simulink model "UAM_Flight_control"  (R2024b)
settings: Solver=FixedStepAuto  StartTime=0.0  StopTime=inf  RelTol=1e-3  EnableMultiTasking=on
undefined symbols (not defined in the file): CityMission, control, controlParams, ControlSampleTime, Cruise_a, DiscIntNeverNeededParam, Earth, FixedWingMission, flightState, FSState, FWControlParams, FWTrimSpeed, HoverMission, params, position, R_WAYPOINTTRANSITION, TransitionMission, uavParam, Vt, w_trim, WGS84, zGround
libraries: slpidlib x56, simulink x35, uavalgslib x8, robotcorelib x2, simulink_extras x2, mspfiltlib x1, aerolibtransform2 x1
(part 1 of 12)
settings Model: DataDictionary=UAM_data.sldd  SimulationMode=external  ExtModeTrigDurationFloating=inf  Creator=admin  LastModifiedBy=USER
settings SolverCC: PositivePriorityOrder=on  AutoInsertRateTranBlk=on
settings OptimizationCC: EnhancedBackFolding=on  PassReuseOutputArgsAs=Individual arguments  ZeroExternalMemoryAtStartup=off  ZeroInternalMemoryAtStartup=off  MaxStackSize=500000  OptimizeBlockOrder=speed  DifferentSizesBufferReuse=on  OptimizationCustomize=off  EfficientTunableParamExpr=on
settings DebuggingCC: ParameterTunabilityLossMsg=error
settings HardwareCC: ProdBitPerLong=64  ProdLargestAtomicInteger=LongLong  ProdLargestAtomicFloat=Double  ProdLongLongMode=on  ProdHWDeviceType=ARM Compatible->ARM Cortex-A (64-bit)
settings ModelReferenceCC: ModelReferenceNumInstancesAllowed=Single
settings SFSimCC: MATLABDynamicMemAlloc=off
settings RTWCC: Description=Embedded Coder  SystemTargetFile=ert.tlc  TemplateMakefile=ert_default_tmf  Toolchain=Linaro AArch64 Linux v6.3.1
settings CodeAppCC: ForceParamTrailComments=on  IgnoreCustomStorageClasses=off  OperatorAnnotations=on  SimulinkDataObjDesc=on  SFDataObjDesc=on  InsertBlockDesc=on
settings ERTTargetCC: TargetLangStandard=C99 (ISO)  ExtModeTransport=1  ExtModeMexFile=ext_serial_win32_comm  InlinedParameterPlacement=Hierarchical  ERTCustomFileTemplate=example_file_process.tlc

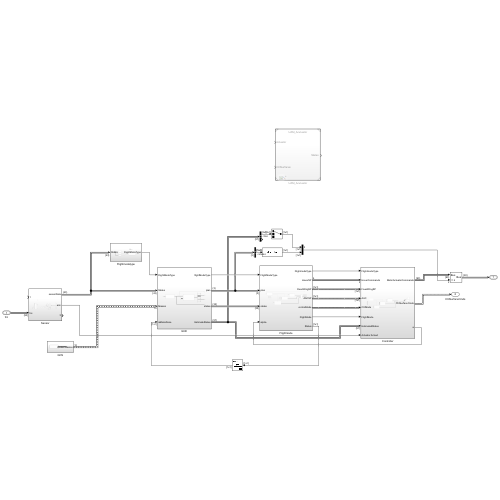
[thumbnail: Simulink's stored preview of the top-level diagram]
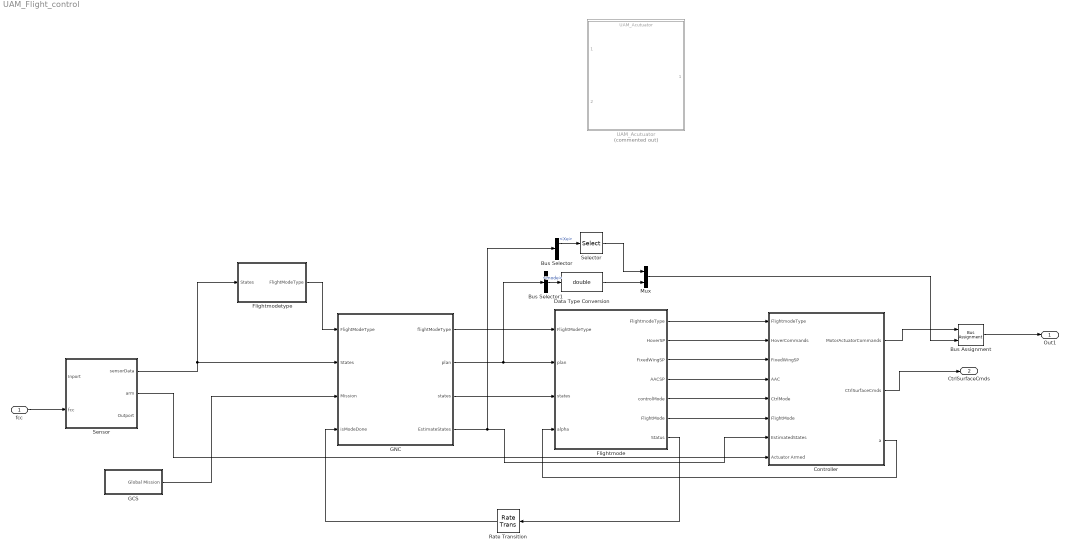
== system UAM_Flight_control ==
  fcc : Inport  OutDataTypeStr=Bus: FCCData
  Bus Assignment : BusAssignment  AssignedSignals=z
  Bus Selector : BusSelector  OutputSignals=Xe,Ve
  Bus Selector1 : BusSelector  OutputSignals=mode
  Controller : Subsystem
  Data Type Conversion : DataTypeConversion  OutDataTypeStr=double  SaturateOnIntegerOverflow=off  RndMeth=Floor
  Flightmode : Subsystem
  Flightmodetype : Subsystem
  GCS : Subsystem
  GNC : Subsystem
  Mux : Mux  Inputs=2
  Rate Transition : RateTransition
  Selector : Selector  InputPortWidth=3  IndexOptions=Index vector (dialog)  Indices=1  OutputSizes=1
  Sensor : Subsystem
  UAM_Acutuator : ModelReference  Commented=on  ModelNameDialog=UAM_Acutuator.slx  SimulationMode=Normal  ModelReferenceVersion=1.21
  Out1 : Outport  OutDataTypeStr=Bus: FCCData  VectorParamsAs1DForOutWhenUnconnected=off
  CtrlSurfaceCmds : Outport  Port=2
  wires:
  Sensor/1(sensorData) -> Flightmodetype/1(States), GNC/2(States)
  GCS/1(Global Mission) -> GNC/3(Mission)
  Flightmodetype/1(FlightModeType) -> GNC/1(FlightModeType)
  GNC/1(flightModeType) -> Flightmode/1(FlightModeType)
  GNC/2(plan) -> Bus Selector1/1, Flightmode/2(plan)
  GNC/3(states) -> Flightmode/3(states)
  Flightmode/1(FlightmodeType) -> Controller/1(FlightmodeType)
  Flightmode/2(HoverSP) -> Controller/2(HoverCommands)
  Flightmode/3(FixedWingSP) -> Controller/3(FixedWingSP)
  Flightmode/4(AACSP) -> Controller/4(AAC)
  Flightmode/5(controlMode) -> Controller/5(CtrlMode)
  Flightmode/6(FlightMode) -> Controller/6(FlightMode)
  GNC/4(EstimateStates) -> Bus Selector/1, Controller/7(EstimatedStates)
  Flightmode/7(Status) -> Rate Transition/1
  Rate Transition/1 -> GNC/4(isModeDone)
  Sensor/2(arm) -> Controller/8(Actuator Armed)
  fcc/1 -> Sensor/2(fcc)
  Controller/3(a) -> Flightmode/4(alpha)
  Controller/2(CtrlSurfaceCmds) -> CtrlSurfaceCmds/1
  Bus Assignment/1 -> Out1/1
  Controller/1(MotorActuatorCommands) -> Bus Assignment/1
  Bus Selector/1 -> Selector/1  "<Xe>"
  Bus Selector1/1 -> Data Type Conversion/1  "<mode>"
  Data Type Conversion/1 -> Mux/2
  Mux/1 -> Bus Assignment/2
  Selector/1 -> Mux/1

== system UAM_Flight_control/Controller ==
  FlightmodeType : Inport  OutDataTypeStr=Enum: FlightModeType
  HoverCommands : Inport  Port=2  OutDataTypeStr=Bus: HoverSPBus
  FixedWingSP : Inport  Port=3  OutDataTypeStr=Bus: FixedWingCommandBus
  AAC : Inport  Port=4  OutDataTypeStr=Bus: AAC
  CtrlMode : Inport  Port=5  OutDataTypeStr=Bus: controlMode
  FlightMode : Inport  Port=6
  EstimatedStates : Inport  Port=7  OutDataTypeStr=Bus: StateBus
  Actuator Armed : Inport  Port=8
  Auto1 : Subsystem  TreatAsAtomicUnit=on
  Bus Selector : BusSelector  OutputSignals=MotorActuatorCommands,CtrlSurfaceCommands,a
  Bus Selector1 : BusSelector  OutputSignals=m
  Bus Selector2 : BusSelector  OutputSignals=rpy_sp
  Display : Display
  Display1 : Display
  Emergency : Subsystem  TreatAsAtomicUnit=on
  Manual : Subsystem  TreatAsAtomicUnit=on
  Merge : Merge  Inputs=3
  Switch Case : SwitchCase  CaseConditions={FlightModeType.Manual, FlightModeType.Auto, FlightModeType.Emergecny}  ShowDefaultCase=off
  MotorActuatorCommands : Outport  OutDataTypeStr=Bus: FCCData
  CtrlSurfaceCmds : Outport  Port=2  OutDataTypeStr=Bus: FixedWingCtrlBus
  a : Outport  Port=3
  wires:
  Bus Selector/3 -> a/1  "<a>"
  [CtrlMode] -> Emergency/1(CtrlMode)
  [CtrlMode] -> Manual/2(CtrlMode)
  AAC/1 -> [AAC]
  [CtrlMode] -> Auto1/4(CtrlMode)
  [FlightMode] -> Emergency/2(FlightMode)
  [EstimatedStates] -> Auto1/6(EstimatedStates)
  Actuator Armed/1 -> [Armed]
  Switch Case/2 -> Auto1/Action
  Bus Selector/2 -> CtrlSurfaceCmds/1  "<CtrlSurfaceCommands>"
  FlightmodeType/1 -> Switch Case/1
  Bus Selector1/1 -> Display/1  "<m>"
  [AAC] -> Auto1/3(AAC)
  CtrlMode/1 -> [CtrlMode]
  Manual/1(Controller) -> Merge/1
  Bus Selector/1 -> Bus Selector2/1, Bus Selector1/1, MotorActuatorCommands/1  "<MotorActuatorCommands>"
  Auto1/1(Controller) -> Merge/2
  Emergency/1(Controller) -> Merge/3
  Switch Case/3 -> Emergency/Action
  Switch Case/1 -> Manual/Action
  [EstimatedStates] -> Manual/4(EstimatedStates)
  [Armed] -> Manual/5(Actuator Armed)
  [FixedWingSP] -> Auto1/2(FixedWingSP)
  FlightMode/1 -> [FlightMode]
  [FlightMode] -> Manual/3(FlightMode)
  FixedWingSP/1 -> [FixedWingSP]
  HoverCommands/1 -> [HoverCommands]
  [EstimatedStates] -> Emergency/3(EstimatedStates)
  [HoverCommands] -> Auto1/1(HoverCommands)
  [Armed] -> Emergency/4(Actuator Armed)
  EstimatedStates/1 -> [EstimatedStates]
  [FlightMode] -> Auto1/5(FlightMode)
  [Armed] -> Auto1/7(" Armed")
  [HoverCommands] -> Manual/1(HoverConmmands)
  Merge/1 -> Bus Selector/1
  Bus Selector2/1 -> Display1/1  "<rpy_sp>"

== system UAM_Flight_control/Flightmode ==
  FlightModeType : Inport
  plan : Inport  Port=2  OutDataTypeStr=Bus: plan
  states : Inport  Port=3  OutDataTypeStr=Bus: states
  alpha : Inport  Port=4
  Auto : Subsystem  TreatAsAtomicUnit=on
  Bus Selector : BusSelector  OutputSignals=HoverSP,FixedWingSP,AACSP,controlMode,FlightMode,Status
  Emergency : Subsystem  TreatAsAtomicUnit=on
  Manual : Subsystem  TreatAsAtomicUnit=on
  Merge : Merge  Inputs=3
  Rate Transition{,1..7} (8 alike) : RateTransition
  Switch Case : SwitchCase  CaseConditions={FlightModeType.Manual, FlightModeType.Auto, FlightModeType.Emergecny}  ShowDefaultCase=off
  Unit Delay : UnitDelay  SampleTime=-1  HasFrameUpgradeWarning=on
  Unit Delay1 : UnitDelay  SampleTime=-1  HasFrameUpgradeWarning=on
  Unit Delay2 : UnitDelay  SampleTime=-1  HasFrameUpgradeWarning=on
  FlightmodeType : Outport  OutDataTypeStr=Enum: FlightModeType
  HoverSP : Outport  Port=2  OutDataTypeStr=Bus: HoverSPBus
  FixedWingSP : Outport  Port=3  OutDataTypeStr=Bus: FixedWingCommandBus
  AACSP : Outport  Port=4  OutDataTypeStr=Bus: AAC
  controlMode : Outport  Port=5  OutDataTypeStr=Bus: controlMode
  FlightMode : Outport  Port=6
  Status : Outport  Port=7
  wires:
  Switch Case/1 -> Manual/Action
  Rate Transition2/1 -> AACSP/1
  [states] -> Manual/1(states)
  Bus Selector/1 -> Rate Transition/1  "<HoverSP>"
  Bus Selector/2 -> Rate Transition1/1  "<FixedWingSP>"
  [alpha] -> Emergency/2(alpha)
  Rate Transition/1 -> HoverSP/1
  [states] -> Emergency/1(states)
  Switch Case/3 -> Emergency/Action
  Rate Transition1/1 -> FixedWingSP/1
  Bus Selector/3 -> Rate Transition2/1  "<AACSP>"
  Bus Selector/5 -> Rate Transition4/1  "<FlightMode>"
  [alpha] -> Manual/2(alpha)
  Rate Transition3/1 -> controlMode/1
  Bus Selector/4 -> Rate Transition3/1  "<controlMode>"
  Bus Selector/6 -> Status/1  "<Status>"
  plan/1 -> Unit Delay/1
  Rate Transition4/1 -> FlightMode/1
  FlightModeType/1 -> FlightmodeType/1, Switch Case/1
  Merge/1 -> Bus Selector/1
  [plan] -> Rate Transition7/1
  [states] -> Rate Transition6/1
  [alpha] -> Rate Transition5/1
  Switch Case/2 -> Auto/Action
  alpha/1 -> Unit Delay2/1
  states/1 -> Unit Delay1/1
  Rate Transition6/1 -> Auto/2(states)
  Rate Transition5/1 -> Auto/3(alpha)
  Rate Transition7/1 -> Auto/1(plan)
  Manual/1(FlightMode) -> Merge/1
  Auto/1(FlightMode) -> Merge/2
  Emergency/1(FlightMode) -> Merge/3
  Unit Delay/1 -> [plan]
  Unit Delay1/1 -> [states]
  Unit Delay2/1 -> [alpha]

== system UAM_Flight_control/Flightmodetype ==
  note: 전환조건
      |
      | 1. ManualInput
      | 2. AutoModeRequest
      | 3. Failsafe
  States : Inport  OutDataTypeStr=Bus: sensorData
  Bus Selector : BusSelector  OutputSignals=RC
  Chart1 : Stateflow chart  TreatAsAtomicUnit=on
      settings: PortSchema="{\"entries\":[{\"content\":{\"sides\":[{\"content\":{\"connectorIds\":[\"In2\",\"In3\",\"In1\"]},\"type\":\"ConnectorPlacement.EquallySpacedRectSide\",\"uuid\":\"7f808d98-1a22-47cf-b619-3081c4328c1f\"},{\"content\":{\"connectorIds\":[\"Out1\"],\"side\":\"RIGHT\"},\"type\":\"ConnectorPlacement.EquallySpacedRectSide\",\"uuid\":\"ee1ebc53-214f-4f44-afa8-7e67f94c306f\"},{\"content\":{\"side\":\"TOP\"},\"type\":\"ConnectorPlacement.EquallySpacedRectSide\",\"uuid\":\"a218192b-9bc0-4f77-b8de-414c3f6a9dd6\"}]},\"type\":\"ConnectorPlacement.EquallySpacedConnector\",\"uuid\":\"d7f6b7da-8a65-4043-9f4e-f6645b75040a\"}],\"packageUris\":[\"http://schema.mathworks.com/mf0/Connector/R2020b\"],\"version\":\"1.0\"}"
  Failsafe : Subsystem
  GCS : Subsystem
  RC : Subsystem
  FlightModeType : Outport  OutDataTypeStr=Enum: FlightModeType
  wires:
  States/1 -> Failsafe/1(States), Bus Selector/1
  Chart1/1(mode) -> FlightModeType/1
  RC/1(ManualInput) -> Chart1/2(ManualInput)
  GCS/1(AutoModeRequest) -> Chart1/3(AutoModeRequest)
  Failsafe/1(Failsafe) -> Chart1/1(Failsafe)
  Bus Selector/1 -> GCS/1(RC_input), RC/1(RCInput)  "<RC>"

== system UAM_Flight_control/GCS ==
  Subsystem : Subsystem
  Global Mission : Outport  OutDataTypeStr=Bus: UAVPathManagerBus  SampleTime=0.005  BusOutputAsStruct=on
  wires:
  Subsystem/1(Mission) -> Global Mission/1

== system UAM_Flight_control/GNC ==
  FlightModeType : Inport  OutDataTypeStr=Enum: FlightModeType
  States : Inport  Port=2  OutDataTypeStr=Bus: sensorData
  Mission : Inport  Port=3  OutDataTypeStr=Bus: UAVPathManagerBus  PortDimensions=10  BusOutputAsStruct=on
  isModeDone : Inport  Port=4  OutDataTypeStr=uint8
  Bus Creator : BusCreator  Inputs=3  OutDataTypeStr=Bus: plan
      settings: InheritFromInputs=off
  Bus Creator1 : BusCreator  Inputs=3  OutDataTypeStr=Bus: states
      settings: InheritFromInputs=off
  Bus Selector : BusSelector  OutputSignals=mode,ToWP,FromWP,pose,states,ground
  Guidance : Subsystem
  Navigation : Subsystem
  flightModeType : Outport
  plan : Outport  Port=2  OutDataTypeStr=Bus: plan
  states : Outport  Port=3  OutDataTypeStr=Bus: states
  EstimateStates : Outport  Port=4  OutDataTypeStr=Bus: StateBus
  wires:
  Mission/1 -> Guidance/3(Mission)
  Bus Selector/6 -> Bus Creator1/3  "<ground>"
  Guidance/1(GNCPlan) -> Bus Selector/1
  Bus Selector/3 -> Bus Creator/3  "<FromWP>"
  Bus Selector/1 -> Bus Creator/1  "<mode>"
  FlightModeType/1 -> Guidance/1(mode), flightModeType/1
  Bus Creator1/1 -> states/1
  Bus Selector/4 -> Bus Creator1/1  "<pose>"
  States/1 -> Navigation/1(sensorData)
  isModeDone/1 -> Guidance/4(isModeDone)
  Bus Selector/2 -> Bus Creator/2  "<ToWP>"
  Bus Selector/5 -> Bus Creator1/2  "<states>"
  Bus Creator/1 -> plan/1
  Navigation/1(States) -> EstimateStates/1, Guidance/2(States)

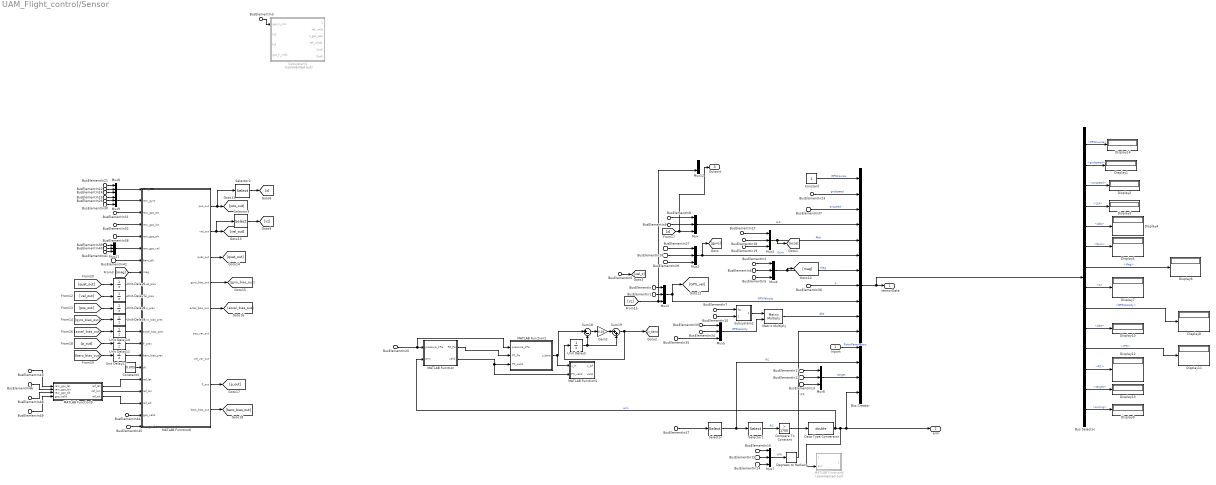
== system UAM_Flight_control/Sensor ==
  Inport : Inport  OutDataTypeStr=Bus: RotorParameters
  BusElementIn14 : Inport  Port=2  PortName=fcc  Element=roll
  BusElementIn15 : Inport  Port=2  PortName=fcc  Element=pitch
  BusElementIn16 : Inport  Port=2  PortName=fcc  Element=yaw
  BusElementIn3 : Inport  Port=2  PortName=fcc  Element=altitude
  BusElementIn8 : Inport  Port=2  PortName=fcc  Element=latitude
  BusElementIn7 : Inport  Port=2  PortName=fcc  Element=latitude
  BusElementIn9 : Inport  Port=2  PortName=fcc  Element=longitude
  BusElementIn10 : Inport  Port=2  PortName=fcc  Element=longitude
  BusElementIn17 : Inport  Port=2  PortName=fcc  Element=acc_x
  BusElementIn18 : Inport  Port=2  PortName=fcc  Element=acc_y
  BusElementIn19 : Inport  Port=2  PortName=fcc  Element=acc_z
  BusElementIn20 : Inport  Port=2  PortName=fcc  Element=pressure
  BusElementIn : Inport  Port=2  PortName=fcc  Element=vel_n
  BusElementIn1 : Inport  Port=2  PortName=fcc  Element=vel_e
  BusElementIn6 : Inport  Port=2  PortName=fcc  Element=vel_d
  BusElementIn23 : Inport  Port=2  PortName=fcc  Element=gndspeed
  BusElementIn11 : Inport  Port=2  PortName=fcc  Element=target_x
  BusElementIn12 : Inport  Port=2  PortName=fcc  Element=target_y
  BusElementIn13 : Inport  Port=2  PortName=fcc  Element=target_z
  BusElementIn27 : Inport  Port=2  PortName=fcc  Element=gyro_x
  BusElementIn28 : Inport  Port=2  PortName=fcc  Element=gyro_y
  BusElementIn29 : Inport  Port=2  PortName=fcc  Element=gyro_z
  BusElementIn2 : Inport  Port=2  PortName=fcc  Element=mag_x
  BusElementIn4 : Inport  Port=2  PortName=fcc  Element=mag_y
  BusElementIn5 : Inport  Port=2  PortName=fcc  Element=mag_z
  BusElementIn33 : Inport  Port=2  PortName=fcc  Element=lin_acc_ecef_x
  BusElementIn34 : Inport  Port=2  PortName=fcc  Element=lin_acc_ecef_y
  BusElementIn35 : Inport  Port=2  PortName=fcc  Element=lin_acc_ecef_z
  BusElementIn36 : Inport  Port=2  PortName=fcc  Element=q
  BusElementIn37 : Inport  Port=2  PortName=fcc  Element=airspeed
  BusElementIn47 : Inport  Port=2  PortName=fcc  Element=rc
  BusElementIn21 : Inport  Port=2  PortName=fcc  Element=raw_acc_x
  BusElementIn22 : Inport  Port=2  PortName=fcc  Element=raw_acc_y
  BusElementIn24 : Inport  Port=2  PortName=fcc  Element=raw_acc_z
  BusElementIn25 : Inport  Port=2  PortName=fcc  Element=raw_gyro_x
  BusElementIn26 : Inport  Port=2  PortName=fcc  Element=raw_gyro_y
  BusElementIn30 : Inport  Port=2  PortName=fcc  Element=raw_gyro_z
  BusElementIn31 : Inport  Port=2  PortName=fcc  Element=raw_gps_lat
  BusElementIn43 : Inport  Port=2  PortName=fcc  Element=raw_gps_lat
  BusElementIn32 : Inport  Port=2  PortName=fcc  Element=raw_gps_lon
  BusElementIn46 : Inport  Port=2  PortName=fcc  Element=raw_gps_lon
  BusElementIn38 : Inport  Port=2  PortName=fcc  Element=raw_gps_alt
  BusElementIn48 : Inport  Port=2  PortName=fcc  Element=raw_gps_alt
  BusElementIn39 : Inport  Port=2  PortName=fcc  Element=raw_vel_n
  BusElementIn40 : Inport  Port=2  PortName=fcc  Element=raw_vel_e
  BusElementIn41 : Inport  Port=2  PortName=fcc  Element=raw_vel_d
  BusElementIn42 : Inport  Port=2  PortName=fcc  Element=baro_alt
  BusElementIn44 : Inport  Port=2  PortName=fcc  Element=gps_valid
  BusElementIn49 : Inport  Port=2  PortName=fcc  Element=gps_valid
  BusElementIn45 : Inport  Port=2  PortName=fcc  Element=baro_valid
  Bus Creator : BusCreator  Inputs=15  OutDataTypeStr=Bus: sensorData
      settings: InheritFromInputs=off
  Bus Selector : BusSelector  OutputSignals=GPSCourse,gndspeed,airspeed,LLA,Abb,Gyro,Mag,q,GPSVelocity,Abe,YPR,RC,target,arming
  Compare To Constant : simulink/Logic and Bit Operations/Compare To Constant  relop=>  const=1700  OutDataTypeStr=boolean
  Constant : Constant
  Constant3 : Constant  Value=0.005
  Data Type Conversion : DataTypeConversion  OutDataTypeStr=double  SaturateOnIntegerOverflow=off  RndMeth=Floor
  Degrees to Radians : simulink_extras/Transformations/Degrees to Radians
  Display{1..14} (14 alike) : Display
  Gain2 : Gain  Gain=0.03
  MATLAB Function : MATLAB Function  TreatAsAtomicUnit=on
  MATLAB Function2 : MATLAB Function  TreatAsAtomicUnit=on
  MATLAB Function5 : MATLAB Function  TreatAsAtomicUnit=on
  MATLAB Function6 : MATLAB Function  Commented=on  TreatAsAtomicUnit=on
  MATLAB Function8 : MATLAB Function  TreatAsAtomicUnit=on  SystemSampleTime=0.005
  MATLAB Function9 : MATLAB Function  TreatAsAtomicUnit=on
  Matrix Multiply : Product  Multiplication=Matrix(*)
  Mux{,1..9,11} (11 alike) : Mux  Inputs=3
  Mux12 : Mux  Inputs=2
  Selector : Selector  InputPortWidth=16  IndexOptions=Index vector (dialog)  Indices=[1:10]  OutputSizes=1
  Selector1 : Selector  InputPortWidth=10  IndexOptions=Index vector (dialog)  Indices=6  OutputSizes=1
  Selector2 : Selector  InputPortWidth=3  IndexOptions=Index vector (dialog)  Indices=3  OutputSizes=1
  Selector3 : Selector  InputPortWidth=3  IndexOptions=Index vector (dialog)  Indices=3  OutputSizes=1
  Subsystem1 : Subsystem  Commented=on
  Subsystem2 : Subsystem
  Sum18 : Sum  Inputs=|+-
  Sum19 : Sum  Inputs=|++
  Unit Delay{6..12} (7 alike) : UnitDelay  SampleTime=-1  HasFrameUpgradeWarning=on
  Unit Delay5 : UnitDelay  SampleTime=0.005  HasFrameUpgradeWarning=on
  sensorData : Outport  OutDataTypeStr=Bus: sensorData
  arm : Outport  Port=2
  Outport : Outport  Port=3
  wires:
  BusElementIn47/1 -> Selector/1
  BusElementIn34/1 -> Mux5/2
  BusElementIn17/1 -> Mux1/1
  Compare To Constant/1 -> Data Type Conversion/1
  Selector/1 -> Bus Creator/13, Selector1/1  "RC"
  BusElementIn4/1 -> Mux4/2
  Subsystem2/1(Out1) -> Matrix Multiply/1
  BusElementIn28/1 -> Mux2/2
  BusElementIn1/1 -> Mux3/2
  BusElementIn9/1 -> Mux/2
  BusElementIn37/1 -> Bus Creator/3  "airspeed"
  BusElementIn35/1 -> Mux5/3
  BusElementIn12/1 -> Mux6/2
  Matrix Multiply/1 -> Bus Creator/10  "Abe"
  BusElementIn27/1 -> Mux2/1
  Selector1/1 -> Compare To Constant/1  "RC"
  Mux5/1 -> Matrix Multiply/2  "GPSVelocity"
  BusElementIn/1 -> Mux3/1
  BusElementIn18/1 -> Mux1/2
  BusElementIn10/1 -> Subsystem2/2(In2)
  BusElementIn36/1 -> Bus Creator/8  "q"
  BusElementIn13/1 -> Mux6/3
  Mux2/1 -> Bus Creator/6, [gyro]  "Gyro"
  BusElementIn7/1 -> Subsystem2/1(fcc)
  Constant/1 -> Bus Creator/1  "GPSCourse"
  BusElementIn2/1 -> Mux4/1
  BusElementIn8/1 -> Mux/1
  Mux/1 -> Bus Creator/4  "LLA"
  BusElementIn33/1 -> Mux5/1
  Data Type Conversion/1 -> MATLAB Function6/2(arm), arm/1, Bus Creator/15, MATLAB Function/2(arm)  "arm"
  Mux4/1 -> [mag], Bus Creator/7  "Mag"
  BusElementIn11/1 -> Mux6/1
  BusElementIn23/1 -> Bus Creator/2  "gndspeed"
  Inport/1 -> Bus Creator/12  "RotorParameters"
  Mux7/1 -> Degrees to Radians/1  "YPR"
  Mux6/1 -> Bus Creator/14  "target"
  BusElementIn16/1 -> Mux7/1
  BusElementIn15/1 -> Mux7/2
  BusElementIn14/1 -> Mux7/3
  Bus Creator/1 -> Bus Selector/1, sensorData/1
  Bus Selector/1 -> Display14/1  "<GPSCourse>"
  Bus Selector/2 -> Display1/1  "<gndspeed>"
  Bus Selector/3 -> Display2/1  "<airspeed>"
  Bus Selector/4 -> Display3/1  "<LLA>"
  Bus Selector/5 -> Display4/1  "<Abb>"
  Bus Selector/6 -> Display5/1  "<Gyro>"
  Bus Selector/7 -> Display6/1  "<Mag>"
  Bus Selector/8 -> Display7/1  "<q>"
  Bus Selector/9 -> Display8/1  "<GPSVelocity>"
  Bus Selector/10 -> Display10/1  "<Abe>"
  Bus Selector/11 -> Display11/1  "<YPR>"
  Bus Selector/12 -> Display12/1  "<RC>"
  Bus Selector/13 -> Display13/1  "<target>"
  Bus Selector/14 -> Display9/1  "<arming>"
  BusElementIn29/1 -> Mux2/3
  BusElementIn5/1 -> Mux4/3
  BusElementIn20/1 -> MATLAB Function2/1(pressure_kPa), MATLAB Function/1(pressure_kPa)
  MATLAB Function/1(P0_Pa) -> MATLAB Function2/2(P0_Pa)
  MATLAB Function/2(valid) -> MATLAB Function5/2(P0_valid), MATLAB Function2/3(P0_valid)
  MATLAB Function2/1(z_baro) -> MATLAB Function5/1(z_in), Sum18/1
  BusElementIn19/1 -> Mux1/3
  Unit Delay5/1 -> Sum19/2, Sum18/2
  Sum18/1 -> Gain2/1
  Gain2/1 -> Sum19/1
  Sum19/1 -> Unit Delay5/1, [z_baro]
  Mux1/1 -> Bus Creator/5, [accel]  "Abb"
  Mux3/1 -> [GPS_vel], Bus Creator/9  "GPSVelocity"
  Degrees to Radians/1 -> Bus Creator/11  "YPR"
  [z] -> Outport/1, Mux/3
  BusElementIn6/1 -> [vel_z]
  [vz] -> Mux12/2, Mux3/3
  BusElementIn21/1 -> Mux8/1
  BusElementIn22/1 -> Mux8/2
  BusElementIn24/1 -> Mux8/3
  Mux8/1 -> MATLAB Function8/1(raw_acc)
  Mux9/1 -> MATLAB Function8/2(raw_gyro)
  BusElementIn25/1 -> Mux9/1
  BusElementIn26/1 -> Mux9/2
  BusElementIn30/1 -> Mux9/3
  BusElementIn31/1 -> MATLAB Function8/3(raw_gps_lat)
  BusElementIn32/1 -> MATLAB Function8/4(raw_gps_lon)
  BusElementIn38/1 -> MATLAB Function8/5(raw_gps_alt)
  BusElementIn39/1 -> Mux11/1
  BusElementIn40/1 -> Mux11/2
  BusElementIn41/1 -> Mux11/3
  Mux11/1 -> MATLAB Function8/6(raw_gps_vel)
  BusElementIn42/1 -> MATLAB Function8/7(baro_alt)
  [mag] -> MATLAB Function8/8(mag)
  BusElementIn44/1 -> MATLAB Function8/20(gps_valid)
  BusElementIn45/1 -> MATLAB Function8/21(baro_valid)
  Constant3/1 -> MATLAB Function8/16(dt)
  Unit Delay6/1 -> MATLAB Function8/9(quat_prev)
  Unit Delay7/1 -> MATLAB Function8/10(vel_prev)
  Unit Delay8/1 -> MATLAB Function8/11(pos_prev)
  Unit Delay9/1 -> MATLAB Function8/12(gyro_bias_prev)
  Unit Delay10/1 -> MATLAB Function8/13(accel_bias_prev)
  Unit Delay11/1 -> MATLAB Function8/14(P_prev)
  Unit Delay12/1 -> MATLAB Function8/15(baro_bias_prev)
  MATLAB Function8/1(pos_out) -> Selector2/1, [pos_out]
  MATLAB Function8/2(vel_out) -> Selector3/1, [vel_out]
  MATLAB Function8/3(quat_out) -> [quat_out]
  MATLAB Function8/4(gyro_bias_out) -> [gyro_bias_out]
  MATLAB Function8/5(accel_bias_out) -> [accel_bias_out]
  MATLAB Function8/8(P_out) -> [p_out]
  MATLAB Function8/9(baro_bias_out) -> [baro_bias_out]
  [vel_out] -> Unit Delay7/1
  [quat_out] -> Unit Delay6/1
  [pos_out] -> Unit Delay8/1
  [gyro_bias_out] -> Unit Delay9/1
  [accel_bias_out] -> Unit Delay10/1
  [p_out] -> Unit Delay11/1
  [baro_bias_out] -> Unit Delay12/1
  MATLAB Function9/1(ref_lat) -> MATLAB Function8/17(ref_lat)
  MATLAB Function9/2(ref_lon) -> MATLAB Function8/18(ref_lon)
  MATLAB Function9/3(ref_alt) -> MATLAB Function8/19(ref_alt)
  BusElementIn43/1 -> MATLAB Function9/1(raw_gps_lat)
  BusElementIn46/1 -> MATLAB Function9/2(raw_gps_lon)
  BusElementIn48/1 -> MATLAB Function9/3(raw_gps_alt)
  BusElementIn49/1 -> MATLAB Function9/4(gps_valid)
  Selector3/1 -> [vz]
  Selector2/1 -> [z]
  BusElementIn3/1 -> Subsystem1/1(gps_h_msl)

== system UAM_Flight_control/Controller/Auto1 ==
  HoverCommands : Inport  OutDataTypeStr=Bus: HoverSPBus
  FixedWingSP : Inport  Port=2
  AAC : Inport  Port=3
  CtrlMode : Inport  Port=4
  FlightMode : Inport  Port=5
  EstimatedStates : Inport  Port=6
  " Armed" : Inport  Port=7
  Action Port : ActionPort  ActionPortLabel=case [ Auto ]:
  Blend Scheduler : Subsystem
  Bus Creator : BusCreator  Inputs=3  OutDataTypeStr=Bus: controller
  Bus Selector2 : BusSelector  OutputSignals=inTransition,TransitionCondition,BackTransitionCondition,TransitionStep
  Fixed Wing Controller : Subsystem  TreatAsAtomicUnit=on  VariantControl=Fixed Wing Controller
  Manual Control : Subsystem
  Multicopter Controller : Subsystem  TreatAsAtomicUnit=on
  Scheduler : Subsystem  SystemSampleTime=0.005
  Controller : Outport
  wires:
  Scheduler/1(MotorActuatorCommands) -> Bus Creator/1  "MotorActuatorCommands"
  Manual Control/1(AERT) -> Fixed Wing Controller/5(AERT)
  Scheduler/2(CtrlSurfaceCommands) -> Bus Creator/2  "CtrlSurfaceCommands"
  Fixed Wing Controller/1(Actuator) -> Scheduler/4(FixedWingActuators)
  Blend Scheduler/2(alpha) -> Bus Creator/3  "a"
  Multicopter Controller/1(MixerCommands) -> Blend Scheduler/3(MixerCommands)
  AAC/1 -> Fixed Wing Controller/3(AAC SP)
  FixedWingSP/1 -> Fixed Wing Controller/4(FixedWingSP)
  [InTransition] -> Multicopter Controller/3(InTransition)
  " Armed"/1 -> Fixed Wing Controller/Enable, Scheduler/Enable, Multicopter Controller/Enable
  HoverCommands/1 -> Multicopter Controller/1(Hover Commands)
  EstimatedStates/1 -> Fixed Wing Controller/1(States), Blend Scheduler/2(States), Multicopter Controller/2(States)
  FlightMode/1 -> Multicopter Controller/5(FlightMode), Blend Scheduler/1(FlightMode)
  Bus Selector2/2 -> [TransitionDone]  "<TransitionCondition>"
  CtrlMode/1 -> Bus Selector2/1, Scheduler/3(CtrlMode), Multicopter Controller/4(CtrlMode), Fixed Wing Controller/2(Control Mode)
  Bus Selector2/1 -> [InTransition]  "<inTransition>"
  Bus Selector2/3 -> [BackTransitionDone]  "<BackTransitionCondition>"
  Bus Creator/1 -> Controller/1
  Blend Scheduler/3(FlightState) -> Scheduler/2(FlightState)
  [InTransition] -> Fixed Wing Controller/6(In1)
  Bus Selector2/4 -> [TransitionStep]  "<TransitionStep>"
  Blend Scheduler/1(MotorCommands) -> Scheduler/1(MotorCommands)

== system UAM_Flight_control/Controller/Emergency ==
  CtrlMode : Inport  OutDataTypeStr=Bus: controlMode
  FlightMode : Inport  Port=2
  EstimatedStates : Inport  Port=3  OutDataTypeStr=Bus: StateBus
  Actuator Armed : Inport  Port=4
  Action Port : ActionPort  ActionPortLabel=case [ Emergecny ]:
  Blend Scheduler : Subsystem
  Bus Creator : BusCreator  Inputs=3  OutDataTypeStr=Bus: controller
  Bus Selector : BusSelector  OutputSignals=TransitionCondition,BackTransitionCondition
  Bus Selector1 : BusSelector  OutputSignals=RC
  Display : Display
  FixedWing Controller : Subsystem  TreatAsAtomicUnit=on  VariantControl=Fixed Wing Controller
  Scheduler : Subsystem  SystemSampleTime=0.005
  multicopter Controller : Subsystem  TreatAsAtomicUnit=on
  Controller : Outport
  wires:
  Blend Scheduler/1(alpha) -> Bus Creator/3, Scheduler/2(BlendingSchedule)  "a"
  [TransitionDone] -> Scheduler/4(TransitionDone)
  EstimatedStates/1 -> FixedWing Controller/1(States), Blend Scheduler/2(States), multicopter Controller/2(States), Bus Selector1/1
  FixedWing Controller/1(Actuator) -> Scheduler/6(FixedWingActuators)
  Bus Selector1/1 -> multicopter Controller/1(RC), FixedWing Controller/3(RC)  "<RC>"
  [BackTransitionDone] -> Scheduler/5(BackTransitionDone)
  Bus Selector/2 -> [BackTransitionDone]  "<BackTransitionCondition>"
  FlightMode/1 -> Blend Scheduler/1(FlightMode)
  Bus Selector/1 -> [TransitionDone]  "<TransitionCondition>"
  Actuator Armed/1 -> Scheduler/Enable, FixedWing Controller/Enable, multicopter Controller/Enable
  CtrlMode/1 -> Bus Selector/1, FixedWing Controller/2(Control Mode)
  Blend Scheduler/2(FlightState) -> Scheduler/3(FlightState)
  multicopter Controller/1(MixerCommands) -> Display/1, Scheduler/1(MotorCommands)
  Scheduler/1(MotorActuatorCommands) -> Bus Creator/1  "MotorActuatorCommands"
  Scheduler/2(CtrlSurfaceCommands) -> Bus Creator/2  "CtrlSurfaceCommands"
  Bus Creator/1 -> Controller/1

== system UAM_Flight_control/Controller/Manual ==
  HoverConmmands : Inport
  CtrlMode : Inport  Port=2  OutDataTypeStr=Bus: controlMode
  FlightMode : Inport  Port=3
  EstimatedStates : Inport  Port=4  OutDataTypeStr=Bus: StateBus
  Actuator Armed : Inport  Port=5
  Action Port : ActionPort  ActionPortLabel=case [ Manual ]:
  Blend Scheduler : Subsystem
  Bus Creator : BusCreator  Inputs=3  OutDataTypeStr=Bus: controller
  Bus Selector : BusSelector  OutputSignals=TransitionCondition,BackTransitionCondition
  Bus Selector1 : BusSelector  OutputSignals=RC
  FixedWing Controller : Subsystem  TreatAsAtomicUnit=on  VariantControl=Fixed Wing Controller
  Scheduler : Subsystem  SystemSampleTime=0.005
  multicopter Controller : Subsystem  TreatAsAtomicUnit=on
  Controller : Outport
  wires:
  Blend Scheduler/1(alpha) -> Bus Creator/3, Scheduler/2(BlendingSchedule)  "a"
  [TransitionDone] -> Scheduler/4(TransitionDone)
  EstimatedStates/1 -> FixedWing Controller/1(States), Blend Scheduler/2(States), multicopter Controller/3(States), Bus Selector1/1
  FixedWing Controller/1(Actuator) -> Scheduler/6(FixedWingActuators)
  Bus Selector1/1 -> FixedWing Controller/3(RC), multicopter Controller/2(RC)  "<RC>"
  [BackTransitionDone] -> Scheduler/5(BackTransitionDone)
  Bus Selector/2 -> [BackTransitionDone]  "<BackTransitionCondition>"
  Bus Selector/1 -> [TransitionDone]  "<TransitionCondition>"
  Actuator Armed/1 -> multicopter Controller/4(arming), Scheduler/Enable, FixedWing Controller/Enable, multicopter Controller/Enable
  CtrlMode/1 -> Bus Selector/1, FixedWing Controller/2(Control Mode)
  Blend Scheduler/2(FlightState) -> Scheduler/3(FlightState)
  multicopter Controller/1(MixerCommands) -> Scheduler/1(MotorCommands)
  Scheduler/1(MotorActuatorCommands) -> Bus Creator/1  "MotorActuatorCommands"
  Scheduler/2(CtrlSurfaceCommands) -> Bus Creator/2  "CtrlSurfaceCommands"
  Bus Creator/1 -> Controller/1
  FlightMode/1 -> Blend Scheduler/1(FlightMode)
  HoverConmmands/1 -> multicopter Controller/1(HoverConmmands)

== system UAM_Flight_control/Flightmode/Auto ==
  plan : Inport  OutDataTypeStr=Bus: plan  SampleTime=0.005
  states : Inport  Port=2  OutDataTypeStr=Bus: states  SampleTime=0.005
  alpha : Inport  Port=3  SampleTime=0.005
  Action Port : ActionPort  ActionPortLabel=case [ Auto ]:
  Bus Creator : BusCreator  Inputs=4  OutDataTypeStr=Bus: HoverSPBus
      settings: InheritFromInputs=off
  Bus Creator1 : BusCreator  Inputs=6  OutDataTypeStr=Bus: flightmode
  Bus Selector : BusSelector  OutputSignals=LAP,YawCmd
  Bus Selector1 : BusSelector  OutputSignals=mode,ToWP,FromWP
  Bus Selector2 : BusSelector  OutputSignals=pose,states,ground
  Compare To Constant : simulink/Logic and Bit Operations/Compare To Constant  relop===  const=2  OutDataTypeStr=boolean
  Constant : Constant  Value=0  OutDataTypeStr=boolean
  Constant2 : Constant  Value=FSState  SampleTime=-1
  Demux : Demux
  Guidance Mode Selector : Stateflow chart  TreatAsAtomicUnit=on
      settings: PortSchema="{\"entries\":[{\"content\":{\"sides\":[{\"content\":{\"connectorIds\":[\"In1\",\"In2\",\"In3\",\"In4\",\"In5\",\"In7\",\"In6\",\"In8\",\"In9\"]},\"type\":\"ConnectorPlacement.EquallySpacedRectSide\",\"uuid\":\"a9cfd0e2-196c-422d-b359-9161a47768c9\"},{\"content\":{\"connectorIds\":[\"Out7\",\"Out2\",\"Out4\",\"Out3\",\"Out5\",\"Out6\",\"Out1\"],\"side\":\"RIGHT\"},\"type\":\"ConnectorPlacement.EquallySpacedRectSide\",\"uuid\":\"4fed41ae-e7cf-4de3-8bdb-9e24e7d8b079\"},{\"content\":{\"side\":\"TOP\"},\"type\":\"ConnectorPlacement.EquallySpacedRectSide\",\"uuid\":\"2d49ff20-2f63-498d-ac9d-820eae01f794\"},{\"content\":{\"side\":\"BOTTOM\"},\"type\":\"ConnectorPlacement.EquallySpacedRectSide\",\"uuid\":\"da24ee44-6e15-4e50-9b36-ff21cb47946d\"}]},\"type\":\"ConnectorPlacement.EquallySpacedConnector\",\"uuid\":\"88d403f4-ad96-40f9-9697-84906f26a8bf\"}],\"packageUris\":[\"http://schema.mathworks.com/mf0/Connector/R2020b\"],\"version\":\"1.0\"}"
  Mux : Mux  Inputs=2
  Stop Simulation : Stop
  Terminator : Terminator
  Unit Delay : UnitDelay  SampleTime=-1  HasFrameUpgradeWarning=on
  FlightMode : Outport  OutDataTypeStr=Bus: flightmode
  wires:
  Bus Selector1/1 -> Guidance Mode Selector/1(mode)  "<mode>"
  Guidance Mode Selector/6(FlightMode) -> Bus Creator1/5  "FlightMode"
  Bus Selector1/3 -> Guidance Mode Selector/3(FromWP)  "<FromWP>"
  Bus Selector2/3 -> Guidance Mode Selector/7(Ground)  "<ground>"
  Bus Selector/1 -> Mux/1  "<LAP>"
  Guidance Mode Selector/5(controlMode) -> Bus Creator1/4  "controlMode"
  Guidance Mode Selector/3(aacSP) -> Bus Creator1/3  "AACSP"
  Guidance Mode Selector/7(InnerLoopCmds) -> Bus Selector/1
  Guidance Mode Selector/2(GdncMode) -> Terminator/1
  Bus Selector/2 -> Mux/2  "<YawCmd>"
  Compare To Constant/1 -> Stop Simulation/1
  Bus Selector2/2 -> Guidance Mode Selector/5(States)  "<states>"
  Mux/1 -> Demux/1
  Bus Selector2/1 -> Guidance Mode Selector/4(Pose)  "<pose>"
  Guidance Mode Selector/1(Status) -> Compare To Constant/1, Bus Creator1/6  "Status"
  Guidance Mode Selector/4(FixedWingSP) -> Bus Creator1/2  "FixedWingSP"
  Bus Selector1/2 -> Guidance Mode Selector/2(ToWP)  "<ToWP>"
  Demux/1 -> Bus Creator/1  "X"
  Demux/2 -> Bus Creator/2  "Y"
  Demux/3 -> Bus Creator/3  "Z"
  Demux/4 -> Bus Creator/4  "Yaw"
  Bus Creator/1 -> Bus Creator1/1  "HoverSP"
  Bus Creator1/1 -> Unit Delay/1
  alpha/1 -> Guidance Mode Selector/8(a)
  Constant2/1 -> Guidance Mode Selector/6(PresetMode)
  states/1 -> Bus Selector2/1
  plan/1 -> Bus Selector1/1
  Unit Delay/1 -> FlightMode/1
  Constant/1 -> Guidance Mode Selector/9(abort_cmd)

== system UAM_Flight_control/Flightmode/Emergency ==
  states : Inport  OutDataTypeStr=Bus: states
  alpha : Inport  Port=2
  Action Port : ActionPort  ActionPortLabel=case [ Emergecny ]:
  Basic Control  Switching : Stateflow chart  TreatAsAtomicUnit=on
  Bus Creator : BusCreator  Inputs=6  OutDataTypeStr=Bus: flightmode
      settings: InheritFromInputs=off
  Bus Creator1 : BusCreator  Inputs=4  OutDataTypeStr=Bus: HoverSPBus
  Bus Selector : BusSelector  OutputSignals=states,states.RC
  Constant{,4..6} (4 alike) : Constant  Value=0
  Constant1 : Constant  Value=struct('roll', 0.0, 'pitch', 0.0, 'yaw', 0.0, 'airspeed', 0.0)  VectorParams1D=off  OutDataTypeStr=Bus: FixedWingCommandBus
  Constant2 : Constant  Value=struct('airspeed', 0.0, 'altitude', 0.0, 'course', 0.0, 'L1', 0.0, 'climbrate', 0.0)  VectorParams1D=off  OutDataTypeStr=Bus: AAC
  Constant3 : Constant  Value=0  OutDataTypeStr=uint8
  Hover : Constant  Value=FSState
  Unit Delay : UnitDelay  SampleTime=-1  HasFrameUpgradeWarning=on
  FlightMode : Outport  OutDataTypeStr=Bus: flightmode
  wires:
  Constant/1 -> Bus Creator1/1  "X"
  Constant5/1 -> Bus Creator1/3  "Z"
  Constant4/1 -> Bus Creator1/2  "Y"
  Basic Control  Switching/2(flightMode) -> Bus Creator/5  "FlightMode"
  Basic Control  Switching/1(controlMode) -> Bus Creator/4  "controlMode"
  Hover/1 -> Basic Control  Switching/1(PresetMode)
  Constant3/1 -> Bus Creator/6  "Status"
  Bus Selector/2 -> Basic Control  Switching/3(trigger)  "<RC>"
  Bus Selector/1 -> Basic Control  Switching/2(States)  "<states>"
  Constant2/1 -> Bus Creator/3  "AACSP"
  alpha/1 -> Basic Control  Switching/4(a)
  Bus Creator1/1 -> Bus Creator/1  "HoverSP"
  states/1 -> Bus Selector/1
  Constant1/1 -> Bus Creator/2  "FixedWingSP"
  Constant6/1 -> Bus Creator1/4  "Yaw"
  Bus Creator/1 -> Unit Delay/1
  Unit Delay/1 -> FlightMode/1

== system UAM_Flight_control/Flightmode/Manual ==
  states : Inport  OutDataTypeStr=Bus: states
  alpha : Inport  Port=2
  Action Port : ActionPort  ActionPortLabel=case [ Manual ]:
  Basic Control  Switching : Stateflow chart  TreatAsAtomicUnit=on
  Bus Creator : BusCreator  Inputs=6  OutDataTypeStr=Bus: flightmode
      settings: InheritFromInputs=off
  Bus Creator1 : BusCreator  Inputs=4  OutDataTypeStr=Bus: HoverSPBus
  Bus Selector : BusSelector  OutputSignals=pose,states,states.RC
  Bus Selector1 : BusSelector  OutputSignals=X,Y,Z,Yaw
  Constant1 : Constant  Value=struct('roll', 0.0, 'pitch', 0.0, 'yaw', 0.0, 'airspeed', 0.0)  VectorParams1D=off  OutDataTypeStr=Bus: FixedWingCommandBus
  Constant2 : Constant  Value=struct('airspeed', 0.0, 'altitude', 0.0, 'course', 0.0, 'L1', 0.0, 'climbrate', 0.0)  VectorParams1D=off  OutDataTypeStr=Bus: AAC
  Constant3 : Constant  Value=0  OutDataTypeStr=uint8
  Display : Display
  Hover : Constant  Value=FSState
  Unit Delay : UnitDelay  SampleTime=-1  HasFrameUpgradeWarning=on
  FlightMode : Outport  OutDataTypeStr=Bus: flightmode
  wires:
  states/1 -> Bus Selector/1
  Basic Control  Switching/2(controlMode) -> Bus Creator/4  "controlMode"
  Hover/1 -> Basic Control  Switching/1(PresetMode)
  Basic Control  Switching/3(flightMode) -> Bus Creator/5  "FlightMode"
  Constant3/1 -> Bus Creator/6  "Status"
  Bus Creator/1 -> Unit Delay/1
  Constant2/1 -> Bus Creator/3  "AACSP"
  Constant1/1 -> Bus Creator/2  "FixedWingSP"
  alpha/1 -> Basic Control  Switching/5(a)
  Bus Selector/2 -> Basic Control  Switching/3(States)  "<states>"
  Bus Selector/3 -> Basic Control  Switching/4(trigger)  "<RC>"
  Unit Delay/1 -> FlightMode/1
  Bus Selector/1 -> Basic Control  Switching/2(pose)  "<pose>"
  Basic Control  Switching/1(HoverSPBUS) -> Bus Selector1/1  "HoverSP"
  Bus Selector1/1 -> Bus Creator1/1  "<X>"
  Bus Selector1/2 -> Bus Creator1/2  "<Y>"
  Bus Selector1/3 -> Bus Creator1/3  "<Z>"
  Bus Selector1/4 -> Bus Creator1/4  "<Yaw>"
  Bus Creator1/1 -> Display/1, Bus Creator/1

== system UAM_Flight_control/Flightmodetype/Failsafe ==
  States : Inport
  Constant : Constant  Value=0
  Data Type Conversion : DataTypeConversion  OutDataTypeStr=boolean  SaturateOnIntegerOverflow=off  RndMeth=Floor
  Failsafe : Outport  OutDataTypeStr=boolean  PortDimensions=1
  wires:
  Constant/1 -> Data Type Conversion/1
  Data Type Conversion/1 -> Failsafe/1

== system UAM_Flight_control/Flightmodetype/GCS ==
  RC_input : Inport
  Compare To Constant : simulink/Logic and Bit Operations/Compare To Constant  relop=>  const=1700  OutDataTypeStr=boolean
  Selector : Selector  InputPortWidth=10  IndexOptions=Index vector (dialog)  Indices=7  OutputSizes=1
  AutoModeRequest : Outport  OutDataTypeStr=boolean
  wires:
  RC_input/1 -> Selector/1
  Selector/1 -> Compare To Constant/1
  Compare To Constant/1 -> AutoModeRequest/1

== system UAM_Flight_control/Flightmodetype/RC ==
  RCInput : Inport
  Compare To Constant : simulink/Logic and Bit Operations/Compare To Constant  relop=<  const=1300  OutDataTypeStr=boolean
  Selector : Selector  InputPortWidth=10  IndexOptions=Index vector (dialog)  Indices=7  OutputSizes=1
  ManualInput : Outport  OutDataTypeStr=boolean
  wires:
  RCInput/1 -> Selector/1
  Compare To Constant/1 -> ManualInput/1
  Selector/1 -> Compare To Constant/1

== system UAM_Flight_control/GCS/Subsystem ==
  note: uavPathManagerBus type
  Airspeed : Constant  Value=16
  Altitude : Constant  Value=0
  Bus Assignment : BusAssignment  AssignedSignals=position,params
  Course : Constant  Value=0
  Flight Mode : Constant  Value=0
  Mux : Mux  Inputs=3
  Mux1 : Mux
  No Mission : Constant  Value=struct('mode',0,'position',[0 0 0]','params',[0;0;0;0]);  OutDataTypeStr=Bus: UAVPathManagerBus
  Variant Source : VariantSource  ShowConditionOnBlock=on
  Waypoints : Constant  Value=FixedWingMission  OutDataTypeStr=Bus: UAVPathManagerBus  SampleTime=-1
  Waypoints1 : Constant  Value=HoverMission  OutDataTypeStr=Bus: UAVPathManagerBus  SampleTime=-1
  Waypoints2 : Constant  Value=TransitionMission  OutDataTypeStr=Bus: UAVPathManagerBus  SampleTime=-1
  Waypoints3 : Constant  Value=CityMission  OutDataTypeStr=Bus: UAVPathManagerBus  SampleTime=-1
  X : Constant  Value=0
  Y : Constant  Value=0
  Z : Constant  Value=10
  Mission : Outport
  wires:
  Waypoints1/1 -> Variant Source/3
  Airspeed/1 -> Mux1/2
  Y/1 -> Mux/2
  No Mission/1 -> Bus Assignment/1
  Z/1 -> Mux/3
  Bus Assignment/1 -> Variant Source/1
  Waypoints/1 -> Variant Source/2
  Flight Mode/1 -> Mux1/1
  X/1 -> Mux/1
  Course/1 -> Mux1/4
  Waypoints3/1 -> Variant Source/5
  Mux/1 -> Bus Assignment/2
  Waypoints2/1 -> Variant Source/4
  Altitude/1 -> Mux1/3
  Mux1/1 -> Bus Assignment/3
  Variant Source/1 -> Mission/1

== system UAM_Flight_control/GNC/Guidance ==
  mode : Inport
  States : Inport  Port=2
  Mission : Inport  Port=3  OutDataTypeStr=Bus: UAVPathManagerBus
  isModeDone : Inport  Port=4
  Atan2 : Trigonometry  Operator=atan2
  Auto : Subsystem  TreatAsAtomicUnit=on
  Bus Selector : BusSelector  OutputSignals=x,y,z,vy,vx
  Emergency : Subsystem  TreatAsAtomicUnit=on
  Merge : Merge  Inputs=3
  Mux : Mux
  Mux1 : Mux  Inputs=2
  Switch Case : SwitchCase  CaseConditions={FlightModeType.Manual, FlightModeType.Auto, FlightModeType.Emergecny}  ShowDefaultCase=off
  Switch Case Action Subsystem : Subsystem  TreatAsAtomicUnit=on
  UAM POS : Subsystem
  UAM States : Subsystem
  ground : Constant  Value=0
  GNCPlan : Outport  OutDataTypeStr=Bus: GNCplan
  wires:
  [pose] -> Emergency/1(pose)
  UAM POS/1(POS) -> Bus Selector/1
  [ground] -> Auto/6(Ground)
  [states] -> Switch Case Action Subsystem/2(states)
  Bus Selector/1 -> Mux/1  "<x>"
  [pose] -> Auto/1(Pose)
  [states] -> Emergency/2(states)
  [isModeDone] -> Auto/3(isModeDone)
  Emergency/1(GNCPlan) -> Merge/3
  [ground] -> Switch Case Action Subsystem/3(ground)
  Auto/1(GNCPlan) -> Merge/2
  [ground] -> Emergency/3(ground)
  Switch Case/1 -> Switch Case Action Subsystem/Action
  Bus Selector/2 -> Mux/2  "<y>"
  [Mission] -> Auto/2(Mission)
  Switch Case Action Subsystem/1(GNCPlan) -> Merge/1
  Atan2/1 -> Mux1/1, Mux/4  "yaw"
  ground/1 -> [ground]
  Merge/1 -> GNCPlan/1
  Switch Case/3 -> Emergency/Action
  [Landingstates] -> Auto/4(LandingStates)
  [states] -> Auto/5(States)
  Bus Selector/3 -> Mux1/2, Mux/3  "<z>"
  [pose] -> Switch Case Action Subsystem/1(pose)
  Switch Case/2 -> Auto/Action
  States/1 -> UAM States/1(UAMStates), UAM POS/1(UAMStates)
  Bus Selector/4 -> Atan2/1  "<vy>"
  Bus Selector/5 -> Atan2/2  "<vx>"
  Mission/1 -> [Mission]
  isModeDone/1 -> [isModeDone]
  UAM States/1(States) -> [states]
  Mux1/1 -> [Landingstates]
  Mux/1 -> [pose]
  mode/1 -> Switch Case/1

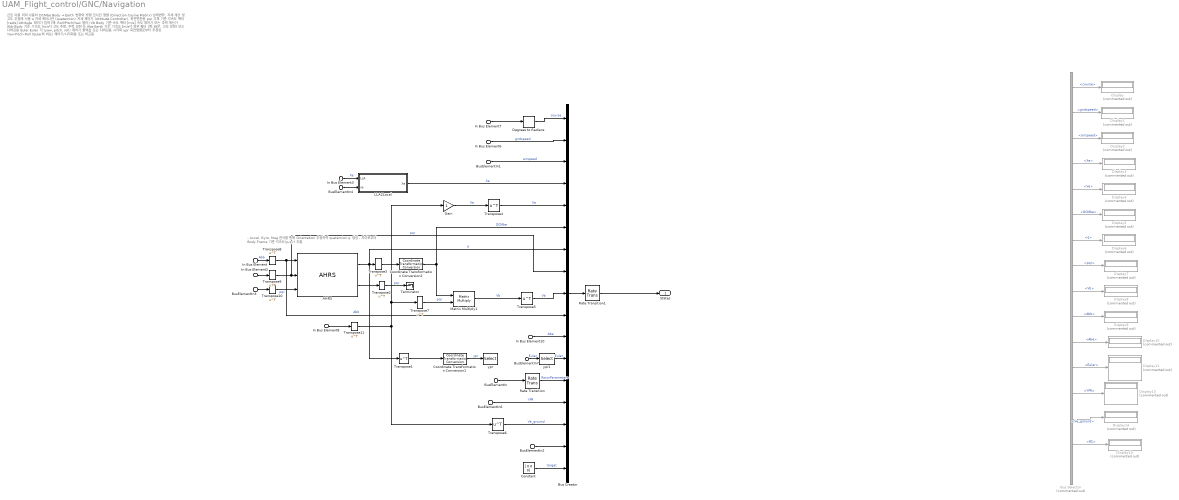
== system UAM_Flight_control/GNC/Navigation ==
  note: 신호 이름
      | 의미
      | 사용처
      |
      | DCMbe
      | Body → Earth 방향의 방향 코사인 행렬 (Direction Cosine Matrix)
      | 상태변환, 자세 계산 및 고도 추정에 사용
      |
      | q
      | 자세 쿼터니언 (quaternion)
      | 자세 제어기 (Attitude Controller), 회전변환용
      |
      | pqr
      | 기체 기준 각속도 벡터 [rad/s]
      | Attitude 제어기 입력 (예: Roll/Pitch/Yaw 제어)
      |
      | Vb
      | Body 기준 속도 벡터 [m/s]
      | 속도 제어기 또는 추력 계산기
      |
      | Abb
      | Body 기준 가속도 [m/s²]
      | 고도 추정, 추력 보정 등
      |
      | Abe
      | Earth 기준 가속도 [m/s²]
      | 외부 필터 (예: EKF, 고도 보정) 또는 디버깅용
      |
      | Euler
      | Euler 각 (yaw, pitch, roll)
      | 제어기 출력값 또는 디버깅용 시각화
      |
      | ypr
      | 회전행렬로부터 추정된 Yaw-Pitch-Roll (Euler와 비슷)
      | 제어기/시각화용 또는 비교용
  note: - Accel, Gyro, Mag 센서를 통해 Orientation 추정하여 quaternion q 생성
      | - 자이로부터 Body Frame 기준 각속도(p,q,r) 추출
  In Bus Element : Inport  PortName=sensorData  Element=Abb
  In Bus Element2 : Inport  PortName=sensorData  Element=Gyro
  In Bus Element3 : Inport  PortName=sensorData  Element=LLA
  In Bus Element6 : Inport  PortName=sensorData  Element=gndspeed
  In Bus Element7 : Inport  PortName=sensorData  Element=GPSCourse
  In Bus Element8 : Inport  PortName=sensorData  Element=GPSVelocity
  In Bus Element10 : Inport  PortName=sensorData  Element=Abe
  BusElementIn : Inport  PortName=sensorData  Element=RotorParameters
  BusElementIn1 : Inport  PortName=sensorData  Element=airspeed
  BusElementIn2 : Inport  PortName=sensorData  Element=RC
  BusElementIn3 : Inport  PortName=sensorData  Element=Mag
  BusElementIn4 : Inport  PortName=sensorData  Element=arming
  BusElementIn6 : Inport  PortName=sensorData  Element=YPR
  BusElementIn7 : Inport  PortName=sensorData  Element=YPR
  AHRS : mspfiltlib/AHRS  DispRefFrame=NED  DecimationFactor=1  InitialProcessNoise=ahrsfilter.defaultProcessNoise  OrientationFormat=quaternion  SimulateUsing=Interpreted execution  AccelerometerNoise=0.0001924722  GyroscopeNoise=9.1385e-5  MagnetometerNoise=0.1  GyroscopeDriftNoise=3.0462e-13  LinearAccelerationNoise=0.0096236100000000012  MagneticDisturbanceNoise=0.5  LinearAccelerationDecayFactor=0.5  MagneticDisturbanceDecayFactor=0.5  ExpectedMagneticFieldStrength=50
  Bus Creator : BusCreator  Inputs=17  OutDataTypeStr=Bus: StateBus
  Bus Selector : BusSelector  Commented=on  OutputSignals=course,gndspeed,airspeed,Xe,Ve,DCMbe,q,pqr,Vb,Abb,Abe,Euler,YPR,Ve_ground,RC,target
  Constant : Constant  Value="[  0 0 0]"
  Coordinate Transformation Conversion1 : robotcorelib/Coordinate Transformation Conversion  InputRepresentation=Quaternion  InputEulerSequence=ZYX  ShowTrVecInputPort=on  OutputRepresentation=Euler Angles  OutputEulerSequence=ZYX  ShowTrVecOutputPort=on  SimulateUsing=Interpreted execution
  Coordinate Transformation Conversion2 : robotcorelib/Coordinate Transformation Conversion  InputRepresentation=Quaternion  InputEulerSequence=ZYX  ShowTrVecInputPort=on  OutputRepresentation=Rotation Matrix  OutputEulerSequence=ZYX  ShowTrVecOutputPort=on  SimulateUsing=Interpreted execution
  Degrees to Radians : simulink_extras/Transformations/Degrees to Radians
  Display{,1..11,13..15} (15 alike) : Display  Commented=on
  Gain : Gain
  LLA2Local : Subsystem
  Matrix Multiply1 : Product  Multiplication=Matrix(*)
  Rate Transition : RateTransition  OutPortSampleTime=0.001
  Rate Transition1 : RateTransition
  Terminator : Terminator
  Transpose{1..11} (11 alike) : Math  Operator=transpose
  ypr : Selector  InputPortWidth=3  IndexOptions=Index vector (dialog)  Indices=[3 2 1]  OutputSizes=1
  ypr1 : Selector  InputPortWidth=3  IndexOptions=Index vector (dialog)  Indices=[3 2 1]  OutputSizes=1
  States : Outport  OutDataTypeStr=Bus: StateBus
  wires:
  Transpose6/1 -> Bus Creator/15  "Ve_ground"
  In Bus Element/1 -> Transpose8/1  "Abb"
  Gain/1 -> Transpose4/1  "Ve"
  In Bus Element8/1 -> Transpose11/1
  Matrix Multiply1/1 -> Transpose5/1  "Vb"
  In Bus Element7/1 -> Degrees to Radians/1
  Rate Transition1/1 -> States/1
  In Bus Element6/1 -> Bus Creator/2  "gndspeed"
  Coordinate Transformation Conversion2/1 -> Bus Creator/6, Matrix Multiply1/1  "DCMbe"
  Transpose5/1 -> Bus Creator/9  "Vb"
  Coordinate Transformation Conversion1/1 -> ypr/1  "ypr"
  In Bus Element10/1 -> Bus Creator/11  "Abe"
  Bus Creator/1 -> Rate Transition1/1
  Rate Transition/1 -> Bus Creator/13  "RotorParameters"
  Degrees to Radians/1 -> Bus Creator/1  "course"
  Transpose4/1 -> Bus Creator/5  "Ve"
  BusElementIn/1 -> Rate Transition/1
  BusElementIn1/1 -> Bus Creator/3  "airspeed"
  BusElementIn2/1 -> Bus Creator/16
  Transpose1/1 -> Coordinate Transformation Conversion1/1
  Transpose3/1 -> Coordinate Transformation Conversion2/1
  Constant/1 -> Bus Creator/17  "target"
  In Bus Element2/1 -> Transpose9/1
  BusElementIn3/1 -> Transpose10/1
  AHRS/1 -> Transpose3/1, Transpose1/1, Bus Creator/7  "q"
  AHRS/2 -> Transpose2/1
  Transpose7/1 -> Matrix Multiply1/2  "pqr"
  Transpose8/1 -> AHRS/1, Bus Creator/10  "Abb"
  Transpose9/1 -> Bus Creator/8, AHRS/2  "pqr"
  Transpose10/1 -> AHRS/3  "pqr"
  Bus Selector/15 -> Display15/1  "<RC>"
  Bus Selector/14 -> Display14/1  "<Ve_ground>"
  Bus Selector/13 -> Display13/1  "<YPR>"
  Bus Selector/12 -> Display11/1  "<Euler>"
  Bus Selector/11 -> Display10/1  "<Abe>"
  Bus Selector/10 -> Display9/1  "<Abb>"
  Bus Selector/9 -> Display8/1  "<Vb>"
  Bus Selector/8 -> Display7/1  "<pqr>"
  Bus Selector/7 -> Display6/1  "<q>"
  Bus Selector/5 -> Display4/1  "<Ve>"
  Bus Selector/4 -> Display3/1  "<Xe>"
  Bus Selector/3 -> Display2/1  "<airspeed>"
  Bus Selector/2 -> Display1/1  "<gndspeed>"
  Bus Selector/6 -> Display5/1  "<DCMbe>"
  Transpose11/1 -> Gain/1, Transpose7/1, Transpose6/1
  BusElementIn6/1 -> Bus Creator/14  "YPR"
  Bus Selector/1 -> Display/1  "<course>"
  BusElementIn7/1 -> ypr1/1  "Euler"
  ypr1/1 -> Bus Creator/12  "Euler"
  Transpose2/1 -> Terminator/1  "pqr"
  BusElementIn4/1 -> LLA2Local/2(ve)
  In Bus Element3/1 -> LLA2Local/1(LLA)  "Xe"
  LLA2Local/1(Xe) -> Bus Creator/4  "Xe"
